simulink model "Offline_SCGAnalysis_2DModCalculator"  (R2019a)
settings: Solver=FixedStepDiscrete  StartTime=0.0  StopTime=param_sim_time  FixedStep=1/fs  MaxStep=1/fs  RelTol=1e-3
undefined symbols (not defined in the file): analyses
settings Model: PacingRate=100  Creator=rcord  LastModifiedBy=rcord
settings SolverCC: ZeroCrossControl=DisableAll
settings DataIOCC: ExternalInput=[t, signals.scg.preprocessing_x, signals.scg.preprocessing_y, signals.scg.preprocessing_z]  LoadExternalInput=on  SignalLogging=off  DSMLogging=off  SaveTime=off  ReturnWorkspaceOutputs=off  TimeSaveName=t_preprocessing  OutputSaveName=out_preprocessing  LoggingIntervals=[-inf,inf]

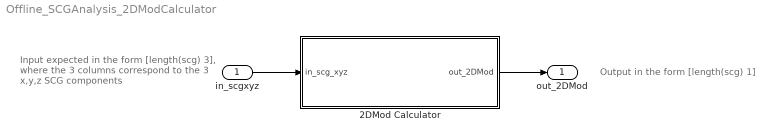
== system Offline_SCGAnalysis_2DModCalculator ==
  note: Output in the form [length(scg) 1]
  note: Input expected in the form [length(scg) 3],
      | where the 3 columns correspond to the
      | 3 x,y,z SCG components
  in_scgxyz : Inport
  2DMod Calculator : Subsystem  mask{xyz2Dcombo=xz (transverse plane)}
      mask prompts: xyz2Dcombo "2D component combination:"
      mask init:
      | if xyz2Dcombo == 1
      |     param_2Dxyzcombo = 'xy';
      | elseif xyz2Dcombo == 2
      |     param_2Dxyzcombo = 'yz';
      | elseif xyz2Dcombo == 3
      |     param_2Dxyzcombo = 'xz';
      | end
      | 
      | assignin('base','param_2Dxyzcombo', param_2Dxyzcombo)
      mask TypeOptions xyz2Dcombo: xy (coronal plane) | yz (sagittal plane) | xz (transverse plane)
      mask DialogControl DescGroupVar Prompt: 2D Modulus Calculator
      mask DialogControl DescTextVar Prompt: Subsystem to calculate a 2D modulus signal from a user-specified combination of any two of the SCG x, y, or z components.
  out_2DMod : Outport
  wires:
  in_scgxyz/1 -> 2DMod Calculator/1(in_scg_xyz)
  2DMod Calculator/1(out_2DMod) -> out_2DMod/1

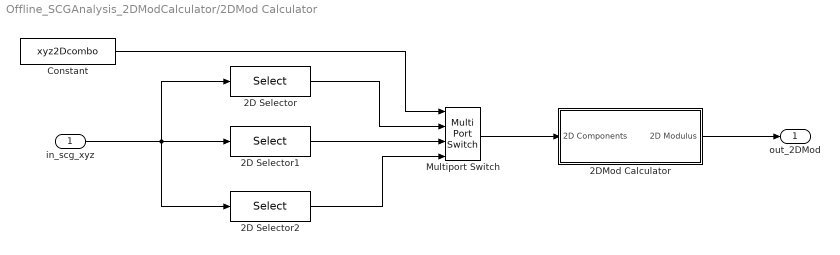
== system Offline_SCGAnalysis_2DModCalculator/2DMod Calculator ==
  in_scg_xyz : Inport
  2D Selector : Selector  NumberOfDimensions=2  IndexOptions=Select all,Index vector (dialog)  Indices=[1:min(analyses.ecg.RR)],[1 2]  OutputSizes=1,1
  2D Selector1 : Selector  NumberOfDimensions=2  IndexOptions=Select all,Index vector (dialog)  Indices=[1:min(analyses.ecg.RR)],[2 3]  OutputSizes=1,1
  2D Selector2 : Selector  NumberOfDimensions=2  IndexOptions=Select all,Index vector (dialog)  Indices=[1:min(analyses.ecg.RR)],[1 3]  OutputSizes=1,1
  2DMod Calculator : Subsystem
  Constant : Constant  Value=xyz2Dcombo
  Multiport Switch : MultiPortSwitch
  out_2DMod : Outport
  wires:
  2DMod Calculator/1(2D Modulus) -> out_2DMod/1
  in_scg_xyz/1 -> 2D Selector2/1, 2D Selector/1, 2D Selector1/1
  Constant/1 -> Multiport Switch/1
  Multiport Switch/1 -> 2DMod Calculator/1(2D Components)
  2D Selector/1 -> Multiport Switch/2
  2D Selector1/1 -> Multiport Switch/3
  2D Selector2/1 -> Multiport Switch/4

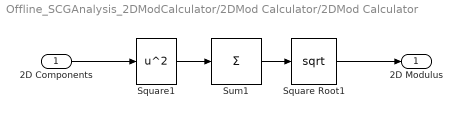
== system Offline_SCGAnalysis_2DModCalculator/2DMod Calculator/2DMod Calculator ==
  2D Components : Inport
  Square Root1 : Sqrt  SaturateOnIntegerOverflow=on
  Square1 : Math  Operator=square  SaturateOnIntegerOverflow=on
  Sum1 : Sum  Inputs=+  CollapseMode=Specified dimension  CollapseDim=2
  2D Modulus : Outport
  wires:
  Square1/1 -> Sum1/1
  Sum1/1 -> Square Root1/1
  2D Components/1 -> Square1/1
  Square Root1/1 -> 2D Modulus/1
